simulink model "euler2GG"  (R2016a)
settings: Solver=VariableStepAuto  StartTime=0.0  StopTime=100000.0  RelTol=1e-3
values from neighbouring files (symbols this model uses):
  Ix = 40    [TestForlineom.m]    (also in TestFornonlineom.m = 30; lineom.m = str2double(get(hObject,'String')); nonlineom.m = str2double(get(hObject,'String')))
  Iy = 50    [TestForlineom.m]    (also in TestFornonlineom.m = 40; lineom.m = str2double(get(hObject,'String')); nonlineom.m = str2double(get(hObject,'String')))
  Iz = 30    [TestForlineom.m]    (also in TestFornonlineom.m = 50; lineom.m = str2double(get(hObject,'String')); nonlineom.m = str2double(get(hObject,'String')))
  phi = 0    [TestForlineom.m]    (also in TestFornonlineom.m = 1.57079632679; lineom.m = str2num(get(hObject,'String')); nonlineom.m = str2num(get(hObject,'String')))
  psi = 0    [TestForlineom.m]    (also in TestFornonlineom.m = 1.57079632679; lineom.m = str2num(get(hObject,'String')); nonlineom.m = str2num(get(hObject,'String')))
  theta = 0.2    [TestForlineom.m]    (also in TestFornonlineom.m = 1.57079632679; lineom.m = str2num(get(hObject,'String')); nonlineom.m = str2num(get(hObject,'String')); saeroanim.m = (360/2/num:360/num:(360+360/2/num))*pi/180)
  Tx = 0    [TestForlineom.m]    (also in lineom.m = str2double(get(hObject,'String')))
  Ty = 0    [TestForlineom.m]    (also in lineom.m = str2double(get(hObject,'String')))
  Tz = 0    [TestForlineom.m]    (also in lineom.m = str2double(get(hObject,'String')))
  w = 2 * pi / (90 * 60)    (= 0.00116355283466)    [TestForlineom.m]    (also in lineom.m = 2 * pi / (tof * 60))
libraries: aerolibanim x1
settings Model: Creator=Mariam Ashraf  LastModifiedBy=shrfm

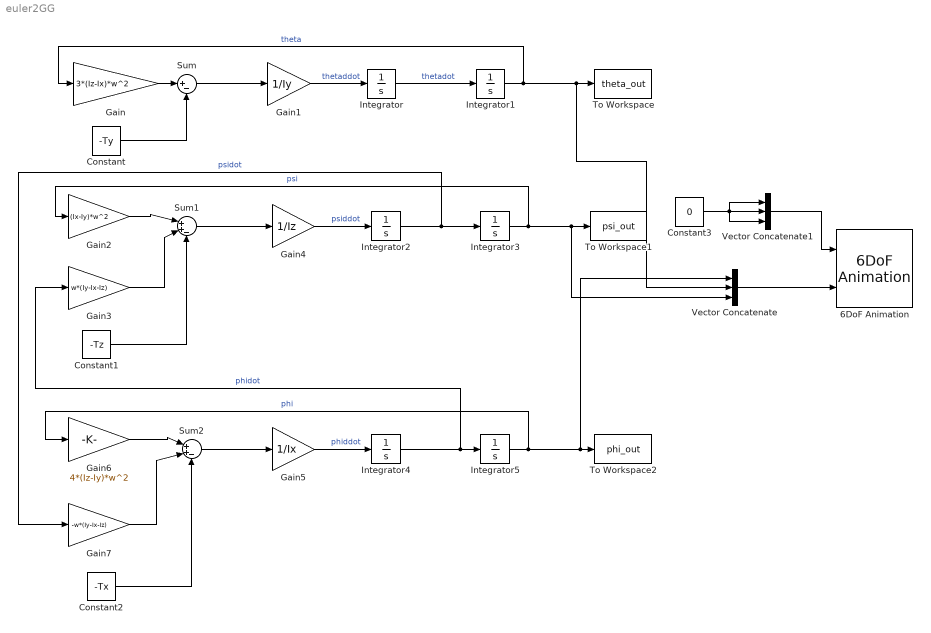
== system euler2GG ==
  6DoF Animation : aerolibanim/6DoF Animation  u1=[0 4000 -2000 2000 -5000 -3000]  u2=100  u3=200  u4=[4000 0 -5000]  u5=Fixed position  u6=[2000 500 -3150]  u7=10  u8=on
  Constant : Constant  Value=-Ty
  Constant1 : Constant  Value=-Tz
  Constant2 : Constant  Value=-Tx
  Constant3 : Constant  Value=0
  Gain : Gain  Gain=3*(Iz-Ix)*w^2
  Gain1 : Gain  Gain=1/Iy
  Gain2 : Gain  Gain=(Ix-Iy)*w^2
  Gain3 : Gain  Gain=w*(Iy-Ix-Iz)
  Gain4 : Gain  Gain=1/Iz
  Gain5 : Gain  Gain=1/Ix
  Gain6 : Gain  Gain=4*(Iz-Iy)*w^2
  Gain7 : Gain  Gain=-w*(Iy-Ix-Iz)
  Integrator : Integrator
  Integrator1 : Integrator  InitialCondition=theta
  Integrator2 : Integrator
  Integrator3 : Integrator  InitialCondition=psi
  Integrator4 : Integrator
  Integrator5 : Integrator  InitialCondition=phi
  Sum : Sum  Inputs=|+-
  Sum1 : Sum  Inputs=|++-
  Sum2 : Sum  Inputs=|++-
  To Workspace : ToWorkspace  VariableName=theta_out  SaveFormat=Timeseries  SampleTime=-1
  To Workspace1 : ToWorkspace  VariableName=psi_out  SaveFormat=Timeseries  SampleTime=-1
  To Workspace2 : ToWorkspace  VariableName=phi_out  SaveFormat=Timeseries  SampleTime=-1
  Vector Concatenate : Concatenate  NumInputs=3
  Vector Concatenate1 : Concatenate  NumInputs=3
  wires:
  Constant/1 -> Sum/2
  Gain/1 -> Sum/1
  Sum/1 -> Gain1/1
  Gain1/1 -> Integrator/1  "thetaddot"
  Integrator/1 -> Integrator1/1  "thetadot"
  Integrator1/1 -> Vector Concatenate/2, To Workspace/1, Gain/1  "theta"
  Gain2/1 -> Sum1/1
  Gain3/1 -> Sum1/2
  Constant1/1 -> Sum1/3
  Sum1/1 -> Gain4/1
  Gain4/1 -> Integrator2/1  "psiddot"
  Integrator2/1 -> Integrator3/1, Gain7/1  "psidot"
  Integrator3/1 -> To Workspace1/1, Vector Concatenate/3, Gain2/1  "psi"
  Gain6/1 -> Sum2/1
  Sum2/1 -> Gain5/1
  Gain5/1 -> Integrator4/1  "phiddot"
  Integrator4/1 -> Gain3/1, Integrator5/1  "phidot"
  Integrator5/1 -> To Workspace2/1, Vector Concatenate/1, Gain6/1  "phi"
  Gain7/1 -> Sum2/2
  Constant2/1 -> Sum2/3
  Vector Concatenate1/1 -> 6DoF Animation/1
  Vector Concatenate/1 -> 6DoF Animation/2
  Constant3/1 -> Vector Concatenate1/3, Vector Concatenate1/1, Vector Concatenate1/2
